simulink model "ImpedanceCtrl_SingleModel"  (R2020b)
settings: Solver=VariableStepAuto  StartTime=0.0  StopTime=50  RelTol=1e-3
undefined symbols (not defined in the file or in its folder): sigbuilder_block
settings Model: Creator=Beta  LastModifiedBy=Beta

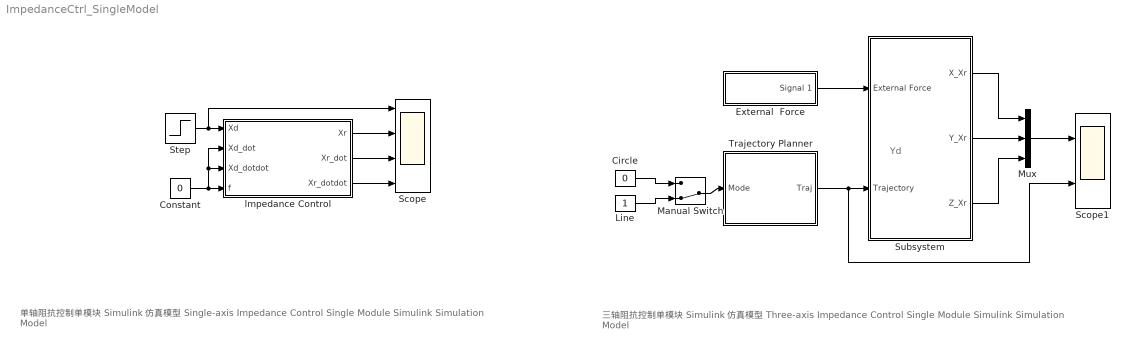
== system ImpedanceCtrl_SingleModel ==
  note: Yd
  note: 单轴阻抗控制单模块 Simulink 仿真模型
      | Single-axis Impedance Control Single Module Simulink Simulation Model
  note: 三轴阻抗控制单模块 Simulink 仿真模型
      | Three-axis Impedance Control Single Module Simulink Simulation Model
  Circle : Constant  Value=0
  Constant : Constant  Value=0
  External  Force : Subsystem  Tag=STV Subsys  LoadFcn=sigbuilder_block('load');  StartFcn=sigbuilder_block('start');  StopFcn=sigbuilder_block('stop');  ClipboardFcn=sigbuilder_block('clipboard');  mask(Sigbuilder block){tuvar=[0:10]}
      mask help: Simulink:masks:SigbuilderBlock_MD
      mask init:
      | if ~strcmp(get_param(bdroot(gcbh),'SimulationStatus'),'stopped') tuvar = sigbuilder_block('maskInit'); end
      settings: CopyFcn=sigbuilder_block('copy');  DeleteFcn=sigbuilder_block('delete');  ModelCloseFcn=sigbuilder_block('modelClose');  PreSaveFcn=sigbuilder_block('preSave');  PauseFcn=sigbuilder_block('pause');  ContinueFcn=sigbuilder_block('continue');  NameChangeFcn=sigbuilder_block('namechange');  OpenFcn=sigbuilder_block('open',[186 132 550.8 400.2 ]);  CloseFcn=sigbuilder_block('close');
      mask Display: plot(0, 0, 100, 100,[2, 2, 32, 32, 2], [68, 8, 8, 68, 68],[32, 2], [38, 38], [32, 19, 2],[53, 60, 44], [32, 17, 17, 2],[16, 16, 31, 31]);txt = getActiveGroup(gcbh);text(2, 100, txt,'verticalAlignment', 'top');
  Line : Constant
  Manual Switch : ManualSwitch  CurrentSetting=0
  Mux : Mux  Inputs=3
  Scope : Scope  NumInputPorts=4
  Scope1 : Scope  NumInputPorts=2
  Step : Step  Time=0  SampleTime=0.005
  Subsystem : Subsystem
  "Trajectory Planner " : Subsystem
      mask Display: image('E:\Traj-tracking Simulation of ER16\3D-Models\image\Trajectory.PNG'); % Use "Edit Image" on toolstrip to change.
  lmpedance Control : MATLAB Function  TreatAsAtomicUnit=on
  wires:
  Constant/1 -> lmpedance Control/4(f), lmpedance Control/3(Xd_dotdot), lmpedance Control/2(Xd_dot)
  Step/1 -> Scope/1, lmpedance Control/1(Xd)
  lmpedance Control/1(Xr) -> Scope/2
  lmpedance Control/2(Xr_dot) -> Scope/3
  lmpedance Control/3(Xr_dotdot) -> Scope/4
  "Trajectory Planner "/1(Traj) -> Scope1/2, Subsystem/2(Trajectory)
  External  Force/1(Signal 1) -> Subsystem/1(External Force)
  Subsystem/1(X_Xr) -> Mux/1
  Subsystem/2(Y_Xr) -> Mux/2
  Subsystem/3(Z_Xr) -> Mux/3
  Mux/1 -> Scope1/1
  Line/1 -> Manual Switch/2
  Manual Switch/1 -> "Trajectory Planner "/1(Mode)
  Circle/1 -> Manual Switch/1

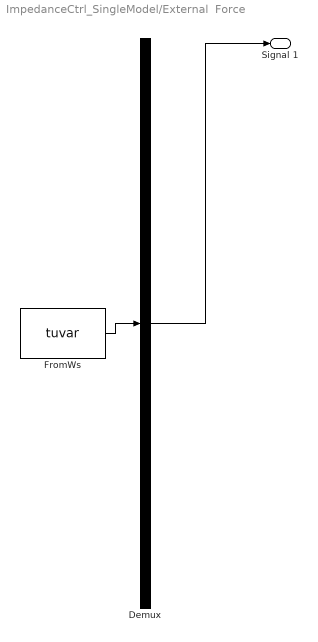
== system ImpedanceCtrl_SingleModel/External  Force ==
  Demux : Demux  Tag=STV Demux  Outputs=1
      settings: DisplayOption=none
  FromWs : FromWorkspace  Tag=STV FromWs  VariableName=tuvar
      SigBuilderData=|
      | common.afterFinalStr = 'Extrapolate'
      | common.sampleTime = 0
      | dataSet.timeRange = [0 50]
      | dataSet.name = 'Group 1'
      | sbobj.Groups.Name = 'Group 1'
      | sbobj.Groups.Signals.Name = 'Signal 1'
      | sbobj.Groups.Signals.XData = [0 15 17 17 35 37 37 50]
      | sbobj.Groups.Signals.YData = [0 -0.005 30 -0.005 0 -30 0 0.5]
      | sbobj.Groups.TimeRange = [0 50]
  Signal 1 : Outport  Tag=STV Outport
  wires:
  Demux/1 -> Signal 1/1
  FromWs/1 -> Demux/1

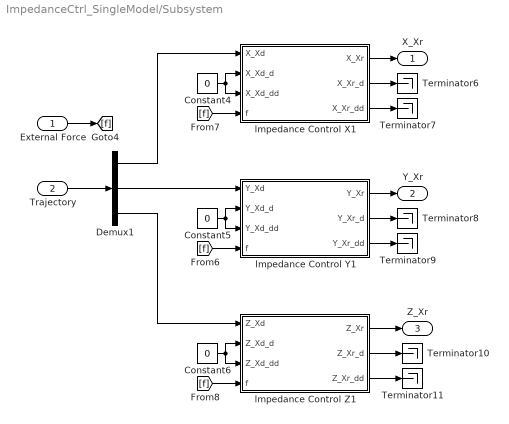
== system ImpedanceCtrl_SingleModel/Subsystem ==
  External Force : Inport
  Trajectory : Inport  Port=2
  Constant4 : Constant  Value=0
  Constant5 : Constant  Value=0
  Constant6 : Constant  Value=0
  Demux1 : Demux  Outputs=3
  Terminator{6..11} (6 alike) : Terminator
  lmpedance Control X1 : MATLAB Function  TreatAsAtomicUnit=on
  lmpedance Control Y1 : MATLAB Function  TreatAsAtomicUnit=on
  lmpedance Control Z1 : MATLAB Function  TreatAsAtomicUnit=on
  X_Xr : Outport
  Y_Xr : Outport  Port=2
  Z_Xr : Outport  Port=3
  wires:
  Trajectory/1 -> Demux1/1
  Constant4/1 -> lmpedance Control X1/3(X_Xd_dd), lmpedance Control X1/2(X_Xd_d)
  External Force/1 -> [f]
  lmpedance Control Y1/3(Y_Xr_dd) -> Terminator9/1
  Demux1/1 -> lmpedance Control X1/1(X_Xd)
  lmpedance Control Y1/1(Y_Xr) -> Y_Xr/1
  Demux1/2 -> lmpedance Control Y1/1(Y_Xd)
  lmpedance Control X1/3(X_Xr_dd) -> Terminator7/1
  Constant6/1 -> lmpedance Control Z1/3(Z_Xd_dd), lmpedance Control Z1/2(Z_Xd_d)
  lmpedance Control X1/1(X_Xr) -> X_Xr/1
  Constant5/1 -> lmpedance Control Y1/3(Y_Xd_dd), lmpedance Control Y1/2(Y_Xd_d)
  lmpedance Control Z1/2(Z_Xr_d) -> Terminator10/1
  [f] -> lmpedance Control Z1/4(f)
  [f] -> lmpedance Control Y1/4(f)
  [f] -> lmpedance Control X1/4(f)
  lmpedance Control Y1/2(Y_Xr_d) -> Terminator8/1
  lmpedance Control X1/2(X_Xr_d) -> Terminator6/1
  lmpedance Control Z1/3(Z_Xr_dd) -> Terminator11/1
  Demux1/3 -> lmpedance Control Z1/1(Z_Xd)
  lmpedance Control Z1/1(Z_Xr) -> Z_Xr/1

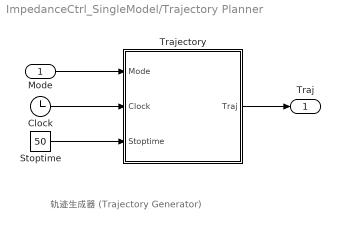
== system ImpedanceCtrl_SingleModel/Trajectory Planner  ==
  note: 轨迹生成器 (Trajectory Generator)
  Mode : Inport
  Clock : Clock
  Stoptime : Constant  Value=50
  Trajectory : MATLAB Function  TreatAsAtomicUnit=on
  Traj : Outport
  wires:
  Trajectory/1(Traj) -> Traj/1
  Clock/1 -> Trajectory/2(Clock)
  Stoptime/1 -> Trajectory/3(Stoptime)
  Mode/1 -> Trajectory/1(Mode)

== matlab function ImpedanceCtrl_SingleModel/lmpedance Control ==
  data: Xd input; Xr output; Xr_dot output; Xr_dotdot output; Xd_dot input; Xd_dotdot input; f input
function [Xr,Xr_dot,Xr_dotdot]  = fcnlmp(Xd,Xd_dot,Xd_dotdot,f)
m =1;b = 4;k=1000;T = 0.005; % 参数初始化
persistent Xr_pre Xr_dot_pre;% 持久变量 https://ww2.mathworks.cn/help/matlab/ref/persistent.html
if isempty(Xr_pre) 
    Xr_pre = 0;
end
if isempty(Xr_dot_pre) 
    Xr_dot_pre = 0;
end
Xr_dotdot_pre = Xd_dotdot + 1/m*(-f + b*(Xd_dot - Xr_dot_pre) + k*(Xd - Xr_pre)); % 上一采样时间 nT 机器人末端的实际运动加速度
Xr = Xr_pre + Xr_dot_pre*T;           % 当前采样时间 (n+1)T 机器人末端的实际运动位置
Xr_dot = Xr_dot_pre + Xr_dotdot_pre*T;% 当前采样时间 (n+1)T 机器人末端的实际运动速度
Xr_dotdot = Xr_dotdot_pre;            % 当前采样时间 (n+1)T 机器人末端的实际运动加速度
Xr_dot_pre = Xr_dot;                  % 上一采样时间 nT 机器人末端的实际运动速度
Xr_pre = Xr;                          % 上一采样时间 nT 机器人末端的实际运动位置
end

== matlab function ImpedanceCtrl_SingleModel/Trajectory Planner /Trajectory ==
  data: Mode input; Traj output; Clock input; Stoptime input
function Traj = traj(Mode,Clock,Stoptime)
    if Mode == 0 % 圆周轨迹
        theta = 2*pi*Clock/Stoptime;
        Xd = 0.2*cos(theta)-0.2;
        Yd = 0;
        Zd = 0.2*sin(theta);
        Traj = [Xd;Yd;Zd];
    else        % 直线轨迹
        Xd = 0;
        Yd = 0;
        Zd = 0.2*Clock/Stoptime;
        Traj = [Xd;Yd;Zd];
    end
end

== matlab function ImpedanceCtrl_SingleModel/Subsystem/lmpedance Control X1 ==
  settings: updateMethod=DISCRETE  sampleTime=0.005
  data: X_Xd input; X_Xr output; X_Xr_d output; X_Xr_dd output; X_Xd_d input; X_Xd_dd input; f input
function [X_Xr,X_Xr_d,X_Xr_dd]  = fcnlmp(X_Xd,X_Xd_d,X_Xd_dd,f)
m =1;b = 200;k=1200;T = 0.005; % 参数初始化
persistent Xr_pre Xr_dot_pre;% 持久变量 https://ww2.mathworks.cn/help/matlab/ref/persistent.html
if isempty(Xr_pre) 
    Xr_pre = 0;
end
if isempty(Xr_dot_pre) 
    Xr_dot_pre = 0;
end
Xr_dotdot_pre = X_Xd_dd + 1/m*(-f + b*(X_Xd_d - Xr_dot_pre) + k*(X_Xd - Xr_pre)); % 上一采样时间 nT 机器人末端的实际运动加速度
X_Xr = Xr_pre + Xr_dot_pre*T;         % 当前采样时间 (n+1)T 机器人末端的实际运动位置
X_Xr_d = Xr_dot_pre + Xr_dotdot_pre*T;% 当前采样时间 (n+1)T 机器人末端的实际运动速度
X_Xr_dd = Xr_dotdot_pre;              % 当前采样时间 (n+1)T 机器人末端的实际运动加速度
Xr_dot_pre = X_Xr_d;                  % 上一采样时间 nT 机器人末端的实际运动速度
Xr_pre = X_Xr;                        % 上一采样时间 nT 机器人末端的实际运动位置
end

== matlab function ImpedanceCtrl_SingleModel/Subsystem/lmpedance Control Y1 ==
  settings: updateMethod=DISCRETE  sampleTime=0.005
  data: Y_Xd input; Y_Xr output; Y_Xr_d output; Y_Xr_dd output; Y_Xd_d input; Y_Xd_dd input; f input
function [Y_Xr,Y_Xr_d,Y_Xr_dd]  = fcnlmp(Y_Xd,Y_Xd_d,Y_Xd_dd,f)
m =1;b = 200;k=1200;T = 0.005; % 参数初始化
persistent Xr_pre Xr_dot_pre;% 持久变量 https://ww2.mathworks.cn/help/matlab/ref/persistent.html
if isempty(Xr_pre) 
    Xr_pre = 0;
end
if isempty(Xr_dot_pre) 
    Xr_dot_pre = 0;
end
Xr_dotdot_pre = Y_Xd_dd + 1/m*(-f + b*(Y_Xd_d - Xr_dot_pre) + k*(Y_Xd - Xr_pre)); % 上一采样时间 nT 机器人末端的实际运动加速度
Y_Xr = Xr_pre + Xr_dot_pre*T;         % 当前采样时间 (n+1)T 机器人末端的实际运动位置
Y_Xr_d = Xr_dot_pre + Xr_dotdot_pre*T;% 当前采样时间 (n+1)T 机器人末端的实际运动速度
Y_Xr_dd = Xr_dotdot_pre;              % 当前采样时间 (n+1)T 机器人末端的实际运动加速度
Xr_dot_pre = Y_Xr_d;                  % 上一采样时间 nT 机器人末端的实际运动速度
Xr_pre = Y_Xr;                        % 上一采样时间 nT 机器人末端的实际运动位置
end

== matlab function ImpedanceCtrl_SingleModel/Subsystem/lmpedance Control Z1 ==
  settings: updateMethod=DISCRETE  sampleTime=0.005
  data: Z_Xd input; Z_Xr output; Z_Xr_d output; Z_Xr_dd output; Z_Xd_d input; Z_Xd_dd input; f input
function [Z_Xr,Z_Xr_d,Z_Xr_dd]  = fcnlmp(Z_Xd,Z_Xd_d,Z_Xd_dd,f)
m =1;b = 200;k=1200;T = 0.005; % 参数初始化
persistent Xr_pre Xr_dot_pre;% 持久变量 https://ww2.mathworks.cn/help/matlab/ref/persistent.html
if isempty(Xr_pre) 
    Xr_pre = 0;
end
if isempty(Xr_dot_pre) 
    Xr_dot_pre = 0;
end
Xr_dotdot_pre = Z_Xd_dd + 1/m*(-f + b*(Z_Xd_d - Xr_dot_pre) + k*(Z_Xd - Xr_pre)); % 上一采样时间 nT 机器人末端的实际运动加速度
Z_Xr = Xr_pre + Xr_dot_pre*T;           % 当前采样时间 (n+1)T 机器人末端的实际运动位置
Z_Xr_d = Xr_dot_pre + Xr_dotdot_pre*T;% 当前采样时间 (n+1)T 机器人末端的实际运动速度
Z_Xr_dd = Xr_dotdot_pre;            % 当前采样时间 (n+1)T 机器人末端的实际运动加速度
Xr_dot_pre = Z_Xr_d;                  % 上一采样时间 nT 机器人末端的实际运动速度
Xr_pre = Z_Xr;                          % 上一采样时间 nT 机器人末端的实际运动位置
end
